simulink model "building_EXAMPLE_v1"  (R2016b)
settings: Solver=ode23tb  StartTime=-building.preruntime+8760*3600  StopTime=building.runtime+8760*3600  MaxStep=600  EnableMultiTasking=on
StartFcn:
  | tic
StopFcn:
  | toc
values from neighbouring files (symbols this model uses):
  building = create_building_automatic(building, modify, import_mode, name_XML, name_EXCEL, name_PHPP, NUMBEROFZONES)    [work_EXAMPLE_v1.m]
undefined symbols (not defined in the file or in its folder): A, B, C, cp, Dd, Dreifach, FluidMix, get_building, ID, MassFlow, p, Pressure, Qdot_C, Qdot_C_energy, Qdot_H, Qdot_H_energy, Qdot_I_electricity, Qdot_I_electricity_energy, Qdot_I_light, Qdot_I_light_energy, Qdot_I_person, Qdot_I_person_energy, Qdot_S, Qdot_S_energy, Qdot_T_ground, Qdot_T_ground_energy, Qdot_T_neighbour, Qdot_T_neighbour_energy, Qdot_T_opaque, Qdot_T_opaque_energy, Qdot_T_window, Qdot_T_window_energy, Qdot_V_infiltration, Qdot_V_infiltration_energy, Qdot_V_mech, Qdot_V_mech_energy, Qdot_V_window, Qdot_V_window_energy, rho, Tc, Temperature, Tr, Ts, Wärmeschutzglas, x_CO2, x_H2O, x_VOC
libraries: carnotUIBK x1931, carnot x83, simulink_extras x22, simulink x12
(part 10 of 35)

== system building_EXAMPLE_v1/DATALOGGER/z2 ==
  BDB : Inport
  BDB_initialize : carnotUIBK/room_node/EMPTY/BDB_initialize
  Bus Assignment : BusAssignment  AssignedSignals=Qdot_T_opaque,Qdot_T_ground,Qdot_T_neighbour,Qdot_T_window,Qdot_V_mech,Qdot_V_window,Qdot_V_infiltration,Qdot_S,Qdot_I_person,Qdot_I_light,Qdot_I_electricity,Qdot_H,Qdot_C
  Bus Selector1 : BusSelector  OutputSignals=Qdot_T_opaque,Qdot_T_ground,Qdot_T_neighbour,Qdot_T_window,Qdot_V_mech,Qdot_V_window,Qdot_V_infiltration,Qdot_S,Qdot_I_person,Qdot_I_light,Qdot_I_electricity,Qdot_H,Qdot_C
  BDB' : Outport
  wires:
  Bus Selector1/2 -> Bus Assignment/3  "<Qdot_T_ground>"
  Bus Selector1/3 -> Bus Assignment/4  "<Qdot_T_neighbour>"
  Bus Selector1/4 -> Bus Assignment/5  "<Qdot_T_window>"
  Bus Selector1/5 -> Bus Assignment/6  "<Qdot_V_mech>"
  Bus Selector1/6 -> Bus Assignment/7  "<Qdot_V_window>"
  Bus Selector1/7 -> Bus Assignment/8  "<Qdot_V_infiltration>"
  Bus Selector1/8 -> Bus Assignment/9  "<Qdot_S>"
  Bus Selector1/9 -> Bus Assignment/10  "<Qdot_I_person>"
  Bus Selector1/10 -> Bus Assignment/11  "<Qdot_I_light>"
  Bus Selector1/11 -> Bus Assignment/12  "<Qdot_I_electricity>"
  Bus Selector1/12 -> Bus Assignment/13  "<Qdot_H>"
  Bus Selector1/13 -> Bus Assignment/14  "<Qdot_C>"
  Bus Selector1/1 -> Bus Assignment/2  "<Qdot_T_opaque>"
  BDB_initialize/1 -> Bus Assignment/1
  Bus Assignment/1 -> BDB'/1
  BDB/1 -> Bus Selector1/1

== system building_EXAMPLE_v1/DATALOGGER/z3 ==
  BDB : Inport
  BDB_initialize : carnotUIBK/room_node/EMPTY/BDB_initialize
  Bus Assignment : BusAssignment  AssignedSignals=Qdot_T_opaque,Qdot_T_ground,Qdot_T_neighbour,Qdot_T_window,Qdot_V_mech,Qdot_V_window,Qdot_V_infiltration,Qdot_S,Qdot_I_person,Qdot_I_light,Qdot_I_electricity,Qdot_H,Qdot_C
  Bus Selector1 : BusSelector  OutputSignals=Qdot_T_opaque,Qdot_T_ground,Qdot_T_neighbour,Qdot_T_window,Qdot_V_mech,Qdot_V_window,Qdot_V_infiltration,Qdot_S,Qdot_I_person,Qdot_I_light,Qdot_I_electricity,Qdot_H,Qdot_C
  BDB' : Outport
  wires:
  BDB/1 -> Bus Selector1/1
  Bus Assignment/1 -> BDB'/1
  BDB_initialize/1 -> Bus Assignment/1
  Bus Selector1/1 -> Bus Assignment/2  "<Qdot_T_opaque>"
  Bus Selector1/13 -> Bus Assignment/14  "<Qdot_C>"
  Bus Selector1/12 -> Bus Assignment/13  "<Qdot_H>"
  Bus Selector1/11 -> Bus Assignment/12  "<Qdot_I_electricity>"
  Bus Selector1/10 -> Bus Assignment/11  "<Qdot_I_light>"
  Bus Selector1/9 -> Bus Assignment/10  "<Qdot_I_person>"
  Bus Selector1/8 -> Bus Assignment/9  "<Qdot_S>"
  Bus Selector1/7 -> Bus Assignment/8  "<Qdot_V_infiltration>"
  Bus Selector1/6 -> Bus Assignment/7  "<Qdot_V_window>"
  Bus Selector1/5 -> Bus Assignment/6  "<Qdot_V_mech>"
  Bus Selector1/4 -> Bus Assignment/5  "<Qdot_T_window>"
  Bus Selector1/3 -> Bus Assignment/4  "<Qdot_T_neighbour>"
  Bus Selector1/2 -> Bus Assignment/3  "<Qdot_T_ground>"

== system building_EXAMPLE_v1/DATALOGGER/z4 ==
  BDB : Inport
  BDB_initialize : carnotUIBK/room_node/EMPTY/BDB_initialize
  Bus Assignment : BusAssignment  AssignedSignals=Qdot_T_opaque,Qdot_T_ground,Qdot_T_neighbour,Qdot_T_window,Qdot_V_mech,Qdot_V_window,Qdot_V_infiltration,Qdot_S,Qdot_I_person,Qdot_I_light,Qdot_I_electricity,Qdot_H,Qdot_C
  Bus Selector1 : BusSelector  OutputSignals=Qdot_T_opaque,Qdot_T_ground,Qdot_T_neighbour,Qdot_T_window,Qdot_V_mech,Qdot_V_window,Qdot_V_infiltration,Qdot_S,Qdot_I_person,Qdot_I_light,Qdot_I_electricity,Qdot_H,Qdot_C
  BDB' : Outport
  wires:
  Bus Selector1/2 -> Bus Assignment/3  "<Qdot_T_ground>"
  Bus Selector1/3 -> Bus Assignment/4  "<Qdot_T_neighbour>"
  Bus Selector1/4 -> Bus Assignment/5  "<Qdot_T_window>"
  Bus Selector1/5 -> Bus Assignment/6  "<Qdot_V_mech>"
  Bus Selector1/6 -> Bus Assignment/7  "<Qdot_V_window>"
  Bus Selector1/7 -> Bus Assignment/8  "<Qdot_V_infiltration>"
  Bus Selector1/8 -> Bus Assignment/9  "<Qdot_S>"
  Bus Selector1/9 -> Bus Assignment/10  "<Qdot_I_person>"
  Bus Selector1/10 -> Bus Assignment/11  "<Qdot_I_light>"
  Bus Selector1/11 -> Bus Assignment/12  "<Qdot_I_electricity>"
  Bus Selector1/12 -> Bus Assignment/13  "<Qdot_H>"
  Bus Selector1/13 -> Bus Assignment/14  "<Qdot_C>"
  Bus Selector1/1 -> Bus Assignment/2  "<Qdot_T_opaque>"
  BDB_initialize/1 -> Bus Assignment/1
  Bus Assignment/1 -> BDB'/1
  BDB/1 -> Bus Selector1/1

== system building_EXAMPLE_v1/DATALOGGER/z5 ==
  BDB : Inport
  BDB_initialize : carnotUIBK/room_node/EMPTY/BDB_initialize
  Bus Assignment : BusAssignment  AssignedSignals=Qdot_T_opaque,Qdot_T_ground,Qdot_T_neighbour,Qdot_T_window,Qdot_V_mech,Qdot_V_window,Qdot_V_infiltration,Qdot_S,Qdot_I_person,Qdot_I_light,Qdot_I_electricity,Qdot_H,Qdot_C
  Bus Selector1 : BusSelector  OutputSignals=Qdot_T_opaque,Qdot_T_ground,Qdot_T_neighbour,Qdot_T_window,Qdot_V_mech,Qdot_V_window,Qdot_V_infiltration,Qdot_S,Qdot_I_person,Qdot_I_light,Qdot_I_electricity,Qdot_H,Qdot_C
  BDB' : Outport
  wires:
  BDB/1 -> Bus Selector1/1
  Bus Assignment/1 -> BDB'/1
  BDB_initialize/1 -> Bus Assignment/1
  Bus Selector1/1 -> Bus Assignment/2  "<Qdot_T_opaque>"
  Bus Selector1/13 -> Bus Assignment/14  "<Qdot_C>"
  Bus Selector1/12 -> Bus Assignment/13  "<Qdot_H>"
  Bus Selector1/11 -> Bus Assignment/12  "<Qdot_I_electricity>"
  Bus Selector1/10 -> Bus Assignment/11  "<Qdot_I_light>"
  Bus Selector1/9 -> Bus Assignment/10  "<Qdot_I_person>"
  Bus Selector1/8 -> Bus Assignment/9  "<Qdot_S>"
  Bus Selector1/7 -> Bus Assignment/8  "<Qdot_V_infiltration>"
  Bus Selector1/6 -> Bus Assignment/7  "<Qdot_V_window>"
  Bus Selector1/5 -> Bus Assignment/6  "<Qdot_V_mech>"
  Bus Selector1/4 -> Bus Assignment/5  "<Qdot_T_window>"
  Bus Selector1/3 -> Bus Assignment/4  "<Qdot_T_neighbour>"
  Bus Selector1/2 -> Bus Assignment/3  "<Qdot_T_ground>"

== system building_EXAMPLE_v1/DATALOGGER/z6 ==
  BDB : Inport
  BDB_initialize : carnotUIBK/room_node/EMPTY/BDB_initialize
  Bus Assignment : BusAssignment  AssignedSignals=Qdot_T_opaque,Qdot_T_ground,Qdot_T_neighbour,Qdot_T_window,Qdot_V_mech,Qdot_V_window,Qdot_V_infiltration,Qdot_S,Qdot_I_person,Qdot_I_light,Qdot_I_electricity,Qdot_H,Qdot_C
  Bus Selector1 : BusSelector  OutputSignals=Qdot_T_opaque,Qdot_T_ground,Qdot_T_neighbour,Qdot_T_window,Qdot_V_mech,Qdot_V_window,Qdot_V_infiltration,Qdot_S,Qdot_I_person,Qdot_I_light,Qdot_I_electricity,Qdot_H,Qdot_C
  BDB' : Outport
  wires:
  Bus Selector1/2 -> Bus Assignment/3  "<Qdot_T_ground>"
  Bus Selector1/3 -> Bus Assignment/4  "<Qdot_T_neighbour>"
  Bus Selector1/4 -> Bus Assignment/5  "<Qdot_T_window>"
  Bus Selector1/5 -> Bus Assignment/6  "<Qdot_V_mech>"
  Bus Selector1/6 -> Bus Assignment/7  "<Qdot_V_window>"
  Bus Selector1/7 -> Bus Assignment/8  "<Qdot_V_infiltration>"
  Bus Selector1/8 -> Bus Assignment/9  "<Qdot_S>"
  Bus Selector1/9 -> Bus Assignment/10  "<Qdot_I_person>"
  Bus Selector1/10 -> Bus Assignment/11  "<Qdot_I_light>"
  Bus Selector1/11 -> Bus Assignment/12  "<Qdot_I_electricity>"
  Bus Selector1/12 -> Bus Assignment/13  "<Qdot_H>"
  Bus Selector1/13 -> Bus Assignment/14  "<Qdot_C>"
  Bus Selector1/1 -> Bus Assignment/2  "<Qdot_T_opaque>"
  BDB_initialize/1 -> Bus Assignment/1
  Bus Assignment/1 -> BDB'/1
  BDB/1 -> Bus Selector1/1

== system building_EXAMPLE_v1/DATALOGGER/z7 ==
  BDB : Inport
  BDB_initialize : carnotUIBK/room_node/EMPTY/BDB_initialize
  Bus Assignment : BusAssignment  AssignedSignals=Qdot_T_opaque,Qdot_T_ground,Qdot_T_neighbour,Qdot_T_window,Qdot_V_mech,Qdot_V_window,Qdot_V_infiltration,Qdot_S,Qdot_I_person,Qdot_I_light,Qdot_I_electricity,Qdot_H,Qdot_C
  Bus Selector1 : BusSelector  OutputSignals=Qdot_T_opaque,Qdot_T_ground,Qdot_T_neighbour,Qdot_T_window,Qdot_V_mech,Qdot_V_window,Qdot_V_infiltration,Qdot_S,Qdot_I_person,Qdot_I_light,Qdot_I_electricity,Qdot_H,Qdot_C
  BDB' : Outport
  wires:
  BDB/1 -> Bus Selector1/1
  Bus Assignment/1 -> BDB'/1
  BDB_initialize/1 -> Bus Assignment/1
  Bus Selector1/1 -> Bus Assignment/2  "<Qdot_T_opaque>"
  Bus Selector1/13 -> Bus Assignment/14  "<Qdot_C>"
  Bus Selector1/12 -> Bus Assignment/13  "<Qdot_H>"
  Bus Selector1/11 -> Bus Assignment/12  "<Qdot_I_electricity>"
  Bus Selector1/10 -> Bus Assignment/11  "<Qdot_I_light>"
  Bus Selector1/9 -> Bus Assignment/10  "<Qdot_I_person>"
  Bus Selector1/8 -> Bus Assignment/9  "<Qdot_S>"
  Bus Selector1/7 -> Bus Assignment/8  "<Qdot_V_infiltration>"
  Bus Selector1/6 -> Bus Assignment/7  "<Qdot_V_window>"
  Bus Selector1/5 -> Bus Assignment/6  "<Qdot_V_mech>"
  Bus Selector1/4 -> Bus Assignment/5  "<Qdot_T_window>"
  Bus Selector1/3 -> Bus Assignment/4  "<Qdot_T_neighbour>"
  Bus Selector1/2 -> Bus Assignment/3  "<Qdot_T_ground>"

== system building_EXAMPLE_v1/DATALOGGER/z8 ==
  BDB : Inport
  BDB_initialize : carnotUIBK/room_node/EMPTY/BDB_initialize
  Bus Assignment : BusAssignment  AssignedSignals=Qdot_T_opaque,Qdot_T_ground,Qdot_T_neighbour,Qdot_T_window,Qdot_V_mech,Qdot_V_window,Qdot_V_infiltration,Qdot_S,Qdot_I_person,Qdot_I_light,Qdot_I_electricity,Qdot_H,Qdot_C
  Bus Selector1 : BusSelector  OutputSignals=Qdot_T_opaque,Qdot_T_ground,Qdot_T_neighbour,Qdot_T_window,Qdot_V_mech,Qdot_V_window,Qdot_V_infiltration,Qdot_S,Qdot_I_person,Qdot_I_light,Qdot_I_electricity,Qdot_H,Qdot_C
  BDB' : Outport
  wires:
  Bus Selector1/2 -> Bus Assignment/3  "<Qdot_T_ground>"
  Bus Selector1/3 -> Bus Assignment/4  "<Qdot_T_neighbour>"
  Bus Selector1/4 -> Bus Assignment/5  "<Qdot_T_window>"
  Bus Selector1/5 -> Bus Assignment/6  "<Qdot_V_mech>"
  Bus Selector1/6 -> Bus Assignment/7  "<Qdot_V_window>"
  Bus Selector1/7 -> Bus Assignment/8  "<Qdot_V_infiltration>"
  Bus Selector1/8 -> Bus Assignment/9  "<Qdot_S>"
  Bus Selector1/9 -> Bus Assignment/10  "<Qdot_I_person>"
  Bus Selector1/10 -> Bus Assignment/11  "<Qdot_I_light>"
  Bus Selector1/11 -> Bus Assignment/12  "<Qdot_I_electricity>"
  Bus Selector1/12 -> Bus Assignment/13  "<Qdot_H>"
  Bus Selector1/13 -> Bus Assignment/14  "<Qdot_C>"
  Bus Selector1/1 -> Bus Assignment/2  "<Qdot_T_opaque>"
  BDB_initialize/1 -> Bus Assignment/1
  Bus Assignment/1 -> BDB'/1
  BDB/1 -> Bus Selector1/1

== system building_EXAMPLE_v1/DATALOGGER/z9 ==
  BDB : Inport
  BDB_initialize : carnotUIBK/room_node/EMPTY/BDB_initialize
  Bus Assignment : BusAssignment  AssignedSignals=Qdot_T_opaque,Qdot_T_ground,Qdot_T_neighbour,Qdot_T_window,Qdot_V_mech,Qdot_V_window,Qdot_V_infiltration,Qdot_S,Qdot_I_person,Qdot_I_light,Qdot_I_electricity,Qdot_H,Qdot_C
  Bus Selector1 : BusSelector  OutputSignals=Qdot_T_opaque,Qdot_T_ground,Qdot_T_neighbour,Qdot_T_window,Qdot_V_mech,Qdot_V_window,Qdot_V_infiltration,Qdot_S,Qdot_I_person,Qdot_I_light,Qdot_I_electricity,Qdot_H,Qdot_C
  BDB' : Outport
  wires:
  BDB/1 -> Bus Selector1/1
  Bus Assignment/1 -> BDB'/1
  BDB_initialize/1 -> Bus Assignment/1
  Bus Selector1/1 -> Bus Assignment/2  "<Qdot_T_opaque>"
  Bus Selector1/13 -> Bus Assignment/14  "<Qdot_C>"
  Bus Selector1/12 -> Bus Assignment/13  "<Qdot_H>"
  Bus Selector1/11 -> Bus Assignment/12  "<Qdot_I_electricity>"
  Bus Selector1/10 -> Bus Assignment/11  "<Qdot_I_light>"
  Bus Selector1/9 -> Bus Assignment/10  "<Qdot_I_person>"
  Bus Selector1/8 -> Bus Assignment/9  "<Qdot_S>"
  Bus Selector1/7 -> Bus Assignment/8  "<Qdot_V_infiltration>"
  Bus Selector1/6 -> Bus Assignment/7  "<Qdot_V_window>"
  Bus Selector1/5 -> Bus Assignment/6  "<Qdot_V_mech>"
  Bus Selector1/4 -> Bus Assignment/5  "<Qdot_T_window>"
  Bus Selector1/3 -> Bus Assignment/4  "<Qdot_T_neighbour>"
  Bus Selector1/2 -> Bus Assignment/3  "<Qdot_T_ground>"

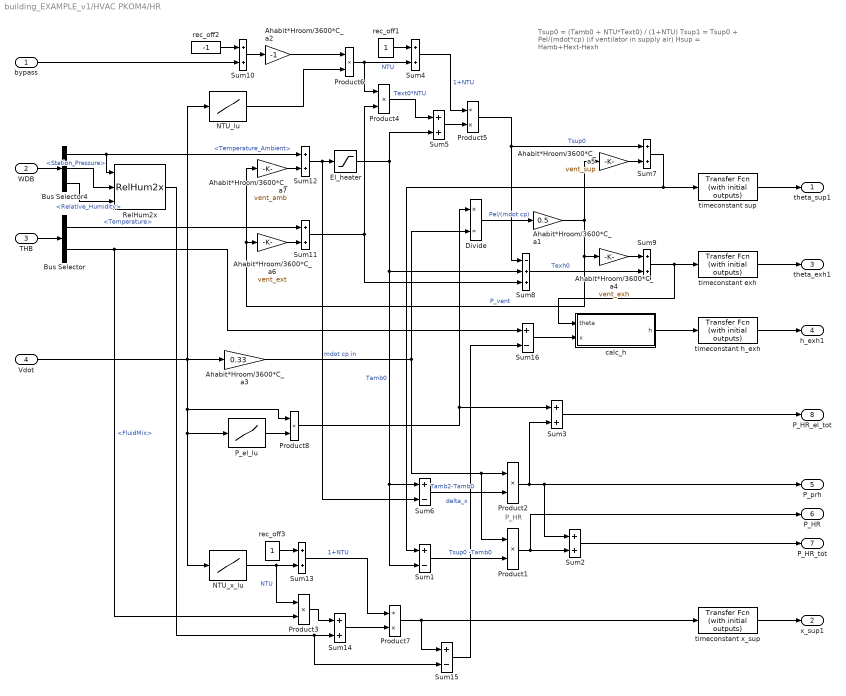
== system building_EXAMPLE_v1/HVAC PKOM4/HR ==
  note: P_HR
  note: Tsup0 = (Tamb0 + NTU*Text0) / (1+NTU)
      | Tsup1 = Tsup0 + Pel/(mdot*cp)  (if ventilator in supply air)
      | Hsup = Hamb+Hext-Hexh
  bypass : Inport
  WDB : Inport  Port=2
  THB : Inport  Port=3
  Vdot : Inport  Port=4
  Ahabit*Hroom/3600*C_a1 : Gain  Gain=0.5  SaturateOnIntegerOverflow=on  OutDataTypeStr=Inherit: Same as input  ParamDataTypeStr=Inherit: Same as input
  Ahabit*Hroom/3600*C_a2 : Gain  Gain=-1  SaturateOnIntegerOverflow=on  OutDataTypeStr=Inherit: Same as input  ParamDataTypeStr=Inherit: Same as input
  Ahabit*Hroom/3600*C_a3 : Gain  Gain=0.33  SaturateOnIntegerOverflow=on  OutDataTypeStr=Inherit: Same as input  ParamDataTypeStr=Inherit: Same as input
  Ahabit*Hroom/3600*C_a4 : Gain  Gain=vent_exh  SaturateOnIntegerOverflow=on  OutDataTypeStr=Inherit: Same as input  ParamDataTypeStr=Inherit: Same as input
  Ahabit*Hroom/3600*C_a5 : Gain  Gain=vent_sup  SaturateOnIntegerOverflow=on  OutDataTypeStr=Inherit: Same as input  ParamDataTypeStr=Inherit: Same as input
  Ahabit*Hroom/3600*C_a6 : Gain  Gain=vent_ext  SaturateOnIntegerOverflow=on  OutDataTypeStr=Inherit: Same as input  ParamDataTypeStr=Inherit: Same as input
  Ahabit*Hroom/3600*C_a7 : Gain  Gain=vent_amb  SaturateOnIntegerOverflow=on  OutDataTypeStr=Inherit: Same as input  ParamDataTypeStr=Inherit: Same as input
  Bus Selector : BusSelector  OutputSignals=Temperature,FluidMix
  Bus Selector4 : BusSelector  OutputSignals=Temperature_Ambient,Station_Pressure,Relative_Humidity
  Divide : Product  Inputs=*/
  El_heater : Saturate  UpperLimit=inf  LowerLimit=low_lim
  NTU_lu : Lookup_n-D  NumberOfTableDimensions=1  BreakpointsForDimension1=Vdot  Table=NTU  InternalRulePriority=Speed  RndMeth=Simplest  InputSameDT=on
  NTU_x_lu : Lookup_n-D  NumberOfTableDimensions=1  BreakpointsForDimension1=Vdot  Table=NTU_x  InternalRulePriority=Speed  RndMeth=Simplest  InputSameDT=on
  P_el_lu : Lookup_n-D  NumberOfTableDimensions=1  BreakpointsForDimension1=Vdot  Table=p_el  InternalRulePriority=Speed  RndMeth=Simplest  InputSameDT=on
  Product{1..4,6,8} (6 alike) : Product  SaturateOnIntegerOverflow=on  InputSameDT=on  OutDataTypeStr=Inherit: Same as first input
  Product5 : Product  Inputs=/*  SaturateOnIntegerOverflow=on  InputSameDT=on  OutDataTypeStr=Inherit: Same as first input
  Product7 : Product  Inputs=/*  SaturateOnIntegerOverflow=on  InputSameDT=on  OutDataTypeStr=Inherit: Same as first input
  RelHum2x : carnot/Basic/Material_Properties/RelHum2x
  Sum{1,6,15..16} (4 alike) : Sum  Inputs=+-  SaturateOnIntegerOverflow=on  InputSameDT=on  OutDataTypeStr=Inherit: Same as first input
  Sum{4..5,7,9..14} (9 alike) : Sum  Inputs=2  SaturateOnIntegerOverflow=on  InputSameDT=on  OutDataTypeStr=Inherit: Same as first input
  Sum2 : Sum  SaturateOnIntegerOverflow=on  InputSameDT=on  OutDataTypeStr=Inherit: Same as first input
  Sum3 : Sum  SaturateOnIntegerOverflow=on  InputSameDT=on  OutDataTypeStr=Inherit: Same as first input
  Sum8 : Sum  Inputs=-++  SaturateOnIntegerOverflow=on  InputSameDT=on  OutDataTypeStr=Inherit: Same as first input
  calc_h : Subsystem
  rec_off1 : Constant
  rec_off2 : Constant  Value=-1
  rec_off3 : Constant
  timeconstant exh : simulink_extras/Additional Linear/Transfer Fcn (with initial outputs)  N=[1]  D=[120 1]  Y0=0  U0=0
  timeconstant h_exh : simulink_extras/Additional Linear/Transfer Fcn (with initial outputs)  N=[1]  D=[120 1]  Y0=0  U0=0
  timeconstant sup : simulink_extras/Additional Linear/Transfer Fcn (with initial outputs)  N=[1]  D=[120 1]  Y0=20  U0=0
  timeconstant x_sup : simulink_extras/Additional Linear/Transfer Fcn (with initial outputs)  N=[1]  D=[120 1]  Y0=0  U0=0
  theta_sup1 : Outport
  x_sup1 : Outport  Port=2
  theta_exh1 : Outport  Port=3
  h_exh1 : Outport  Port=4
  P_prh : Outport  Port=5
  P_HR : Outport  Port=6
  P_HR_tot : Outport  Port=7
  P_HR_el_tot : Outport  Port=8
  wires:
  P_el_lu/1 -> Product8/2
  timeconstant x_sup/1 -> x_sup1/1
  timeconstant h_exh/1 -> h_exh1/1
  timeconstant exh/1 -> theta_exh1/1
  timeconstant sup/1 -> theta_sup1/1
  Sum16/1 -> calc_h/2(x)
  Sum15/1 -> Sum16/2  "delta_x"
  Product7/1 -> Sum15/1, timeconstant x_sup/1
  Sum14/1 -> Product7/2
  Product3/1 -> Sum14/1
  NTU_x_lu/1 -> Sum13/2, Product3/1  "NTU"
  Sum13/1 -> Product7/1  "1+NTU"
  rec_off3/1 -> Sum13/1
  Bus Selector4/3 -> RelHum2x/3  "<Relative_Humidity>"
  Bus Selector4/2 -> RelHum2x/2  "<Station_Pressure>"
  RelHum2x/1 -> Sum14/2, Sum15/2
  Sum6/1 -> Product2/2  "Tamb2-Tamb0"
  Sum9/1 -> calc_h/1(theta), timeconstant exh/1
  Sum11/1 -> Sum8/3, Product4/2
  Vdot/1 -> Ahabit*Hroom/3600*C_a3/1, NTU_lu/1, NTU_x_lu/1, P_el_lu/1, Product8/1
  Sum7/1 -> timeconstant sup/1, Sum1/1
  El_heater/1 -> Sum5/2, Sum6/1, Sum1/2, Sum8/2  "Tamb0"
  Product2/1 -> P_prh/1, Sum2/1, Sum3/2
  Sum1/1 -> Product1/2  "Tsup0 -Tamb0"
  Product1/1 -> Sum2/2, P_HR/1
  Sum2/1 -> P_HR_tot/1
  Sum3/1 -> P_HR_el_tot/1
  Product6/1 -> Product4/1, Sum4/2  "NTU"
  NTU_lu/1 -> Product6/2
  Sum4/1 -> Product5/1  "1+NTU"
  Product4/1 -> Sum5/1  "Text0*NTU"
  rec_off1/1 -> Sum4/1
  Sum5/1 -> Product5/2
  Product5/1 -> Sum7/1, Sum8/1  "Tsup0"
  Divide/1 -> Ahabit*Hroom/3600*C_a1/1  "Pel/(mdot cp)"
  Product8/1 -> Sum3/1, Divide/1
  Ahabit*Hroom/3600*C_a1/1 -> Ahabit*Hroom/3600*C_a5/1, Ahabit*Hroom/3600*C_a7/1, Ahabit*Hroom/3600*C_a6/1, Ahabit*Hroom/3600*C_a4/1  "P_vent"
  Sum8/1 -> Sum9/2  "Texh0"
  Ahabit*Hroom/3600*C_a3/1 -> Divide/2, Product2/1, Product1/1  "mdot cp in"
  Ahabit*Hroom/3600*C_a2/1 -> Product6/1
  rec_off2/1 -> Sum10/1
  bypass/1 -> Sum10/2
  Sum10/1 -> Ahabit*Hroom/3600*C_a2/1
  WDB/1 -> Bus Selector4/1
  Sum12/1 -> El_heater/1, Sum6/2
  THB/1 -> Bus Selector/1
  Ahabit*Hroom/3600*C_a4/1 -> Sum9/1
  Ahabit*Hroom/3600*C_a5/1 -> Sum7/2
  calc_h/1(h) -> timeconstant h_exh/1
  Bus Selector/2 -> Product3/2, Sum16/1  "<FluidMix>"
  Ahabit*Hroom/3600*C_a6/1 -> Sum11/2
  Bus Selector/1 -> Sum11/1  "<Temperature>"
  Ahabit*Hroom/3600*C_a7/1 -> Sum12/2
  Bus Selector4/1 -> Sum12/1, RelHum2x/1  "<Temperature_Ambient>"

== system building_EXAMPLE_v1/HVAC PKOM4/HR unit ==
  note: P_HR
  note: Tsup0 = (Tamb0 + NTU*Text0) / (1+NTU)
      | Tsup1 = Tsup0 + Pel/(mdot*cp)  (if ventilator in supply air)
      | Hsup = Hamb+Hext-Hexh
  bypass : Inport
  WDB : Inport  Port=2
  THB : Inport  Port=3
  Vdot : Inport  Port=4
  Ahabit*Hroom/3600*C_a1 : Gain  Gain=0.5  SaturateOnIntegerOverflow=on  OutDataTypeStr=Inherit: Same as input  ParamDataTypeStr=Inherit: Same as input
  Ahabit*Hroom/3600*C_a2 : Gain  Gain=-1  SaturateOnIntegerOverflow=on  OutDataTypeStr=Inherit: Same as input  ParamDataTypeStr=Inherit: Same as input
  Ahabit*Hroom/3600*C_a3 : Gain  Gain=cp_a * rho_a / 3600  SaturateOnIntegerOverflow=on  OutDataTypeStr=Inherit: Same as input  ParamDataTypeStr=Inherit: Same as input
  Ahabit*Hroom/3600*C_a4 : Gain  Gain=vent_exh  SaturateOnIntegerOverflow=on  OutDataTypeStr=Inherit: Same as input  ParamDataTypeStr=Inherit: Same as input
  Ahabit*Hroom/3600*C_a5 : Gain  Gain=vent_sup  SaturateOnIntegerOverflow=on  OutDataTypeStr=Inherit: Same as input  ParamDataTypeStr=Inherit: Same as input
  Ahabit*Hroom/3600*C_a6 : Gain  Gain=vent_ext  SaturateOnIntegerOverflow=on  OutDataTypeStr=Inherit: Same as input  ParamDataTypeStr=Inherit: Same as input
  Ahabit*Hroom/3600*C_a7 : Gain  Gain=vent_amb  SaturateOnIntegerOverflow=on  OutDataTypeStr=Inherit: Same as input  ParamDataTypeStr=Inherit: Same as input
  Bus Selector : BusSelector  OutputSignals=Temperature,FluidMix
  Bus Selector4 : BusSelector  OutputSignals=Temperature_Ambient,Station_Pressure,Relative_Humidity
  Divide : Product  Inputs=*/
  El_heater : Saturate  UpperLimit=inf  LowerLimit=low_lim
  NTU : Constant  Value=NTU
  Product{1..2,4,6} (4 alike) : Product  SaturateOnIntegerOverflow=on  InputSameDT=on  OutDataTypeStr=Inherit: Same as first input
  Product5 : Product  Inputs=/*  SaturateOnIntegerOverflow=on  InputSameDT=on  OutDataTypeStr=Inherit: Same as first input
  RelHum2x : carnot/Basic/Material_Properties/RelHum2x
  Sum1 : Sum  Inputs=+-  SaturateOnIntegerOverflow=on  InputSameDT=on  OutDataTypeStr=Inherit: Same as first input
  Sum{4..5,7,9..12} (7 alike) : Sum  Inputs=2  SaturateOnIntegerOverflow=on  InputSameDT=on  OutDataTypeStr=Inherit: Same as first input
  Sum2 : Sum  SaturateOnIntegerOverflow=on  InputSameDT=on  OutDataTypeStr=Inherit: Same as first input
  Sum3 : Sum  SaturateOnIntegerOverflow=on  InputSameDT=on  OutDataTypeStr=Inherit: Same as first input
  Sum6 : Sum  Inputs=+-  SaturateOnIntegerOverflow=on  InputSameDT=on  OutDataTypeStr=Inherit: Same as first input
  Sum8 : Sum  Inputs=-++  SaturateOnIntegerOverflow=on  InputSameDT=on  OutDataTypeStr=Inherit: Same as first input
  calc_h : Subsystem
  rec_off1 : Constant
  rec_off2 : Constant  Value=-1
  rec_off4 : Constant  Value=P_elec
  theta_sup1 : Outport
  x_sup1 : Outport  Port=2
  theta_exh1 : Outport  Port=3
  h_exh1 : Outport  Port=4
  P_prh : Outport  Port=5
  P_HR : Outport  Port=6
  P_HR_tot : Outport  Port=7
  P_HR_el_tot : Outport  Port=8
  wires:
  Sum6/1 -> Product2/2  "Tamb2-Tamb0"
  Sum9/1 -> calc_h/1(theta), theta_exh1/1
  Sum11/1 -> Sum8/3, Product4/2
  Vdot/1 -> Ahabit*Hroom/3600*C_a3/1
  Sum7/1 -> theta_sup1/1, Sum1/1
  El_heater/1 -> Sum6/1, Sum1/2, Sum8/2, Sum5/2  "Tamb0"
  Product2/1 -> P_prh/1, Sum2/1, Sum3/2
  Sum1/1 -> Product1/2  "Tsup0 -Tamb0"
  Product1/1 -> Sum2/2, P_HR/1
  Sum2/1 -> P_HR_tot/1
  Sum3/1 -> P_HR_el_tot/1
  Product6/1 -> Product4/1, Sum4/2  "NTU"
  NTU/1 -> Product6/2
  Sum4/1 -> Product5/1  "1+NTU"
  Product4/1 -> Sum5/1  "Text0*NTU"
  rec_off1/1 -> Sum4/1
  Sum5/1 -> Product5/2
  Product5/1 -> Sum7/1, Sum8/1  "Tsup0"
  Divide/1 -> Ahabit*Hroom/3600*C_a1/1  "Pel/(mdot cp)"
  rec_off4/1 -> Sum3/1, Divide/1
  Ahabit*Hroom/3600*C_a1/1 -> Ahabit*Hroom/3600*C_a5/1, Ahabit*Hroom/3600*C_a7/1, Ahabit*Hroom/3600*C_a6/1, Ahabit*Hroom/3600*C_a4/1  "P_vent"
  Sum8/1 -> Sum9/2  "Texh0"
  Ahabit*Hroom/3600*C_a3/1 -> Divide/2, Product2/1, Product1/1  "mdot cp in"
  Ahabit*Hroom/3600*C_a2/1 -> Product6/1
  rec_off2/1 -> Sum10/1
  bypass/1 -> Sum10/2
  Sum10/1 -> Ahabit*Hroom/3600*C_a2/1
  WDB/1 -> Bus Selector4/1
  Sum12/1 -> El_heater/1, Sum6/2
  THB/1 -> Bus Selector/1
  Ahabit*Hroom/3600*C_a4/1 -> Sum9/1
  Ahabit*Hroom/3600*C_a5/1 -> Sum7/2
  calc_h/1(h) -> h_exh1/1
  Bus Selector/2 -> calc_h/2(x)  "<FluidMix>"
  Ahabit*Hroom/3600*C_a6/1 -> Sum11/2
  Bus Selector/1 -> Sum11/1  "<Temperature>"
  Ahabit*Hroom/3600*C_a7/1 -> Sum12/2
  Bus Selector4/1 -> Sum12/1, RelHum2x/1  "<Temperature_Ambient>"
  Bus Selector4/2 -> RelHum2x/2  "<Station_Pressure>"
  Bus Selector4/3 -> RelHum2x/3  "<Relative_Humidity>"
  RelHum2x/1 -> x_sup1/1

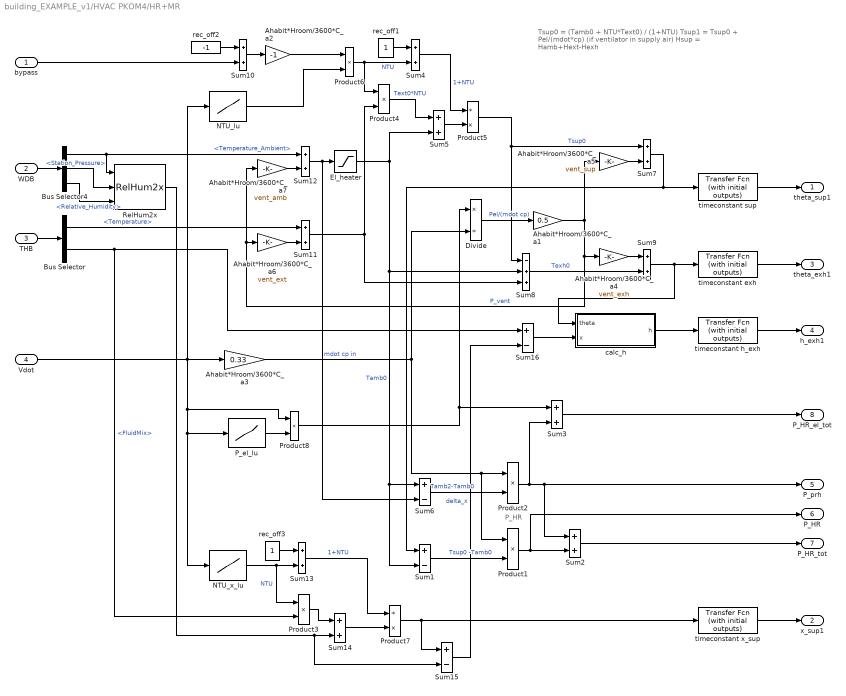
== system building_EXAMPLE_v1/HVAC PKOM4/HR+MR ==
  note: Tsup0 = (Tamb0 + NTU*Text0) / (1+NTU)
      | Tsup1 = Tsup0 + Pel/(mdot*cp)  (if ventilator in supply air)
      | Hsup = Hamb+Hext-Hexh
  note: P_HR
  bypass : Inport
  WDB : Inport  Port=2
  THB : Inport  Port=3
  Vdot : Inport  Port=4
  Ahabit*Hroom/3600*C_a1 : Gain  Gain=0.5  SaturateOnIntegerOverflow=on  OutDataTypeStr=Inherit: Same as input  ParamDataTypeStr=Inherit: Same as input
  Ahabit*Hroom/3600*C_a2 : Gain  Gain=-1  SaturateOnIntegerOverflow=on  OutDataTypeStr=Inherit: Same as input  ParamDataTypeStr=Inherit: Same as input
  Ahabit*Hroom/3600*C_a3 : Gain  Gain=0.33  SaturateOnIntegerOverflow=on  OutDataTypeStr=Inherit: Same as input  ParamDataTypeStr=Inherit: Same as input
  Ahabit*Hroom/3600*C_a4 : Gain  Gain=vent_exh  SaturateOnIntegerOverflow=on  OutDataTypeStr=Inherit: Same as input  ParamDataTypeStr=Inherit: Same as input
  Ahabit*Hroom/3600*C_a5 : Gain  Gain=vent_sup  SaturateOnIntegerOverflow=on  OutDataTypeStr=Inherit: Same as input  ParamDataTypeStr=Inherit: Same as input
  Ahabit*Hroom/3600*C_a6 : Gain  Gain=vent_ext  SaturateOnIntegerOverflow=on  OutDataTypeStr=Inherit: Same as input  ParamDataTypeStr=Inherit: Same as input
  Ahabit*Hroom/3600*C_a7 : Gain  Gain=vent_amb  SaturateOnIntegerOverflow=on  OutDataTypeStr=Inherit: Same as input  ParamDataTypeStr=Inherit: Same as input
  Bus Selector : BusSelector  OutputSignals=Temperature,FluidMix
  Bus Selector4 : BusSelector  OutputSignals=Temperature_Ambient,Station_Pressure,Relative_Humidity
  Divide : Product  Inputs=*/
  El_heater : Saturate  UpperLimit=inf  LowerLimit=low_lim
  NTU_lu : Lookup_n-D  NumberOfTableDimensions=1  BreakpointsForDimension1=Vdot  Table=NTU  InternalRulePriority=Speed  RndMeth=Simplest  InputSameDT=on
  NTU_x_lu : Lookup_n-D  NumberOfTableDimensions=1  BreakpointsForDimension1=Vdot  Table=NTU_x  InternalRulePriority=Speed  RndMeth=Simplest  InputSameDT=on
  P_el_lu : Lookup_n-D  NumberOfTableDimensions=1  BreakpointsForDimension1=Vdot  Table=p_el  InternalRulePriority=Speed  RndMeth=Simplest  InputSameDT=on
  Product{1..4,6,8} (6 alike) : Product  SaturateOnIntegerOverflow=on  InputSameDT=on  OutDataTypeStr=Inherit: Same as first input
  Product5 : Product  Inputs=/*  SaturateOnIntegerOverflow=on  InputSameDT=on  OutDataTypeStr=Inherit: Same as first input
  Product7 : Product  Inputs=/*  SaturateOnIntegerOverflow=on  InputSameDT=on  OutDataTypeStr=Inherit: Same as first input
  RelHum2x : carnot/Basic/Material_Properties/RelHum2x
  Sum{1,6,15..16} (4 alike) : Sum  Inputs=+-  SaturateOnIntegerOverflow=on  InputSameDT=on  OutDataTypeStr=Inherit: Same as first input
  Sum{4..5,7,9..14} (9 alike) : Sum  Inputs=2  SaturateOnIntegerOverflow=on  InputSameDT=on  OutDataTypeStr=Inherit: Same as first input
  Sum2 : Sum  SaturateOnIntegerOverflow=on  InputSameDT=on  OutDataTypeStr=Inherit: Same as first input
  Sum3 : Sum  SaturateOnIntegerOverflow=on  InputSameDT=on  OutDataTypeStr=Inherit: Same as first input
  Sum8 : Sum  Inputs=-++  SaturateOnIntegerOverflow=on  InputSameDT=on  OutDataTypeStr=Inherit: Same as first input
  calc_h : Subsystem
  rec_off1 : Constant
  rec_off2 : Constant  Value=-1
  rec_off3 : Constant
  timeconstant exh : simulink_extras/Additional Linear/Transfer Fcn (with initial outputs)  N=[1]  D=[120 1]  Y0=0  U0=0
  timeconstant h_exh : simulink_extras/Additional Linear/Transfer Fcn (with initial outputs)  N=[1]  D=[120 1]  Y0=0  U0=0
  timeconstant sup : simulink_extras/Additional Linear/Transfer Fcn (with initial outputs)  N=[1]  D=[120 1]  Y0=20  U0=0
  timeconstant x_sup : simulink_extras/Additional Linear/Transfer Fcn (with initial outputs)  N=[1]  D=[120 1]  Y0=0  U0=0
  theta_sup1 : Outport
  x_sup1 : Outport  Port=2
  theta_exh1 : Outport  Port=3
  h_exh1 : Outport  Port=4
  P_prh : Outport  Port=5
  P_HR : Outport  Port=6
  P_HR_tot : Outport  Port=7
  P_HR_el_tot : Outport  Port=8
  wires:
  Bus Selector4/1 -> RelHum2x/1, Sum12/1  "<Temperature_Ambient>"
  Ahabit*Hroom/3600*C_a7/1 -> Sum12/2
  Bus Selector/1 -> Sum11/1  "<Temperature>"
  Ahabit*Hroom/3600*C_a6/1 -> Sum11/2
  Bus Selector/2 -> Sum16/1, Product3/2  "<FluidMix>"
  calc_h/1(h) -> timeconstant h_exh/1
  Ahabit*Hroom/3600*C_a5/1 -> Sum7/2
  Ahabit*Hroom/3600*C_a4/1 -> Sum9/1
  THB/1 -> Bus Selector/1
  Sum12/1 -> Sum6/2, El_heater/1
  WDB/1 -> Bus Selector4/1
  Sum10/1 -> Ahabit*Hroom/3600*C_a2/1
  bypass/1 -> Sum10/2
  rec_off2/1 -> Sum10/1
  Ahabit*Hroom/3600*C_a2/1 -> Product6/1
  Ahabit*Hroom/3600*C_a3/1 -> Product1/1, Product2/1, Divide/2  "mdot cp in"
  Sum8/1 -> Sum9/2  "Texh0"
  Ahabit*Hroom/3600*C_a1/1 -> Ahabit*Hroom/3600*C_a4/1, Ahabit*Hroom/3600*C_a6/1, Ahabit*Hroom/3600*C_a7/1, Ahabit*Hroom/3600*C_a5/1  "P_vent"
  Product8/1 -> Divide/1, Sum3/1
  Divide/1 -> Ahabit*Hroom/3600*C_a1/1  "Pel/(mdot cp)"
  Product5/1 -> Sum8/1, Sum7/1  "Tsup0"
  Sum5/1 -> Product5/2
  rec_off1/1 -> Sum4/1
  Product4/1 -> Sum5/1  "Text0*NTU"
  Sum4/1 -> Product5/1  "1+NTU"
  NTU_lu/1 -> Product6/2
  Product6/1 -> Sum4/2, Product4/1  "NTU"
  Sum3/1 -> P_HR_el_tot/1
  Sum2/1 -> P_HR_tot/1
  Product1/1 -> P_HR/1, Sum2/2
  Sum1/1 -> Product1/2  "Tsup0 -Tamb0"
  Product2/1 -> Sum3/2, Sum2/1, P_prh/1
  El_heater/1 -> Sum8/2, Sum1/2, Sum6/1, Sum5/2  "Tamb0"
  Sum7/1 -> Sum1/1, timeconstant sup/1
  Vdot/1 -> Product8/1, P_el_lu/1, NTU_x_lu/1, NTU_lu/1, Ahabit*Hroom/3600*C_a3/1
  Sum11/1 -> Product4/2, Sum8/3
  Sum9/1 -> timeconstant exh/1, calc_h/1(theta)
  Sum6/1 -> Product2/2  "Tamb2-Tamb0"
  RelHum2x/1 -> Sum15/2, Sum14/2
  Bus Selector4/2 -> RelHum2x/2  "<Station_Pressure>"
  Bus Selector4/3 -> RelHum2x/3  "<Relative_Humidity>"
  rec_off3/1 -> Sum13/1
  Sum13/1 -> Product7/1  "1+NTU"
  NTU_x_lu/1 -> Product3/1, Sum13/2  "NTU"
  Product3/1 -> Sum14/1
  Sum14/1 -> Product7/2
  Product7/1 -> timeconstant x_sup/1, Sum15/1
  Sum15/1 -> Sum16/2  "delta_x"
  Sum16/1 -> calc_h/2(x)
  timeconstant sup/1 -> theta_sup1/1
  timeconstant exh/1 -> theta_exh1/1
  timeconstant h_exh/1 -> h_exh1/1
  timeconstant x_sup/1 -> x_sup1/1
  P_el_lu/1 -> Product8/2

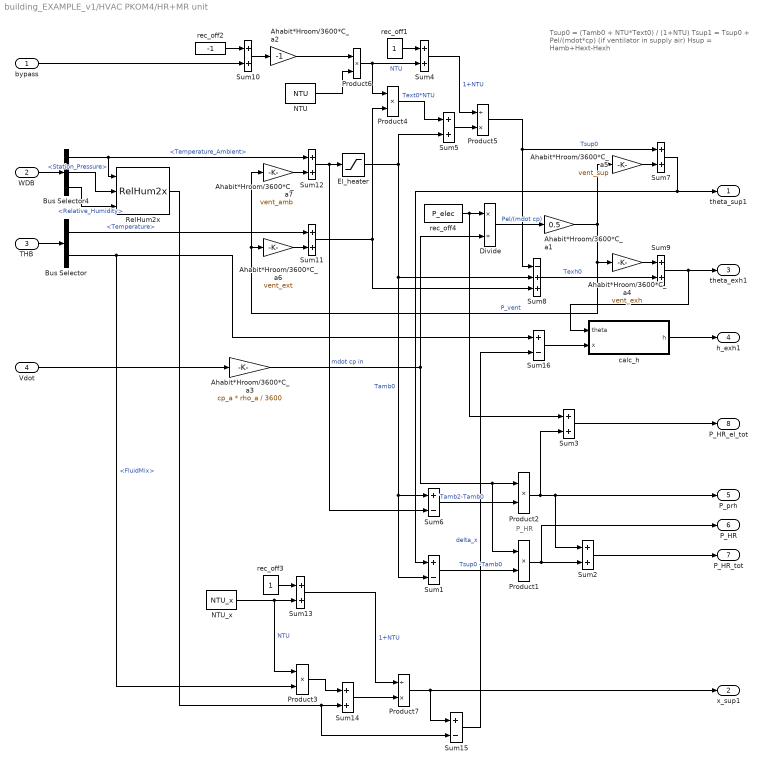
== system building_EXAMPLE_v1/HVAC PKOM4/HR+MR unit ==
  note: Tsup0 = (Tamb0 + NTU*Text0) / (1+NTU)
      | Tsup1 = Tsup0 + Pel/(mdot*cp)  (if ventilator in supply air)
      | Hsup = Hamb+Hext-Hexh
  note: P_HR
  bypass : Inport
  WDB : Inport  Port=2
  THB : Inport  Port=3
  Vdot : Inport  Port=4
  Ahabit*Hroom/3600*C_a1 : Gain  Gain=0.5  SaturateOnIntegerOverflow=on  OutDataTypeStr=Inherit: Same as input  ParamDataTypeStr=Inherit: Same as input
  Ahabit*Hroom/3600*C_a2 : Gain  Gain=-1  SaturateOnIntegerOverflow=on  OutDataTypeStr=Inherit: Same as input  ParamDataTypeStr=Inherit: Same as input
  Ahabit*Hroom/3600*C_a3 : Gain  Gain=cp_a * rho_a / 3600  SaturateOnIntegerOverflow=on  OutDataTypeStr=Inherit: Same as input  ParamDataTypeStr=Inherit: Same as input
  Ahabit*Hroom/3600*C_a4 : Gain  Gain=vent_exh  SaturateOnIntegerOverflow=on  OutDataTypeStr=Inherit: Same as input  ParamDataTypeStr=Inherit: Same as input
  Ahabit*Hroom/3600*C_a5 : Gain  Gain=vent_sup  SaturateOnIntegerOverflow=on  OutDataTypeStr=Inherit: Same as input  ParamDataTypeStr=Inherit: Same as input
  Ahabit*Hroom/3600*C_a6 : Gain  Gain=vent_ext  SaturateOnIntegerOverflow=on  OutDataTypeStr=Inherit: Same as input  ParamDataTypeStr=Inherit: Same as input
  Ahabit*Hroom/3600*C_a7 : Gain  Gain=vent_amb  SaturateOnIntegerOverflow=on  OutDataTypeStr=Inherit: Same as input  ParamDataTypeStr=Inherit: Same as input
  Bus Selector : BusSelector  OutputSignals=Temperature,FluidMix
  Bus Selector4 : BusSelector  OutputSignals=Temperature_Ambient,Station_Pressure,Relative_Humidity
  Divide : Product  Inputs=*/
  El_heater : Saturate  UpperLimit=inf  LowerLimit=low_lim
  NTU : Constant  Value=NTU
  NTU_x : Constant  Value=NTU_x
  Product{1..4,6} (5 alike) : Product  SaturateOnIntegerOverflow=on  InputSameDT=on  OutDataTypeStr=Inherit: Same as first input
  Product5 : Product  Inputs=/*  SaturateOnIntegerOverflow=on  InputSameDT=on  OutDataTypeStr=Inherit: Same as first input
  Product7 : Product  Inputs=/*  SaturateOnIntegerOverflow=on  InputSameDT=on  OutDataTypeStr=Inherit: Same as first input
  RelHum2x : carnot/Basic/Material_Properties/RelHum2x
  Sum{1,6,15..16} (4 alike) : Sum  Inputs=+-  SaturateOnIntegerOverflow=on  InputSameDT=on  OutDataTypeStr=Inherit: Same as first input
  Sum{4..5,7,9..14} (9 alike) : Sum  Inputs=2  SaturateOnIntegerOverflow=on  InputSameDT=on  OutDataTypeStr=Inherit: Same as first input
  Sum2 : Sum  SaturateOnIntegerOverflow=on  InputSameDT=on  OutDataTypeStr=Inherit: Same as first input
  Sum3 : Sum  SaturateOnIntegerOverflow=on  InputSameDT=on  OutDataTypeStr=Inherit: Same as first input
  Sum8 : Sum  Inputs=-++  SaturateOnIntegerOverflow=on  InputSameDT=on  OutDataTypeStr=Inherit: Same as first input
  calc_h : Subsystem
  rec_off1 : Constant
  rec_off2 : Constant  Value=-1
  rec_off3 : Constant
  rec_off4 : Constant  Value=P_elec
  theta_sup1 : Outport
  x_sup1 : Outport  Port=2
  theta_exh1 : Outport  Port=3
  h_exh1 : Outport  Port=4
  P_prh : Outport  Port=5
  P_HR : Outport  Port=6
  P_HR_tot : Outport  Port=7
  P_HR_el_tot : Outport  Port=8
  wires:
  Bus Selector4/1 -> RelHum2x/1, Sum12/1  "<Temperature_Ambient>"
  Ahabit*Hroom/3600*C_a7/1 -> Sum12/2
  Bus Selector/1 -> Sum11/1  "<Temperature>"
  Ahabit*Hroom/3600*C_a6/1 -> Sum11/2
  Bus Selector/2 -> Sum16/1, Product3/2  "<FluidMix>"
  calc_h/1(h) -> h_exh1/1
  Ahabit*Hroom/3600*C_a5/1 -> Sum7/2
  Ahabit*Hroom/3600*C_a4/1 -> Sum9/1
  THB/1 -> Bus Selector/1
  Sum12/1 -> Sum6/2, El_heater/1
  WDB/1 -> Bus Selector4/1
  Sum10/1 -> Ahabit*Hroom/3600*C_a2/1
  bypass/1 -> Sum10/2
  rec_off2/1 -> Sum10/1
  Ahabit*Hroom/3600*C_a2/1 -> Product6/1
  Ahabit*Hroom/3600*C_a3/1 -> Product1/1, Product2/1, Divide/2  "mdot cp in"
  Sum8/1 -> Sum9/2  "Texh0"
  Ahabit*Hroom/3600*C_a1/1 -> Ahabit*Hroom/3600*C_a4/1, Ahabit*Hroom/3600*C_a6/1, Ahabit*Hroom/3600*C_a7/1, Ahabit*Hroom/3600*C_a5/1  "P_vent"
  rec_off4/1 -> Divide/1, Sum3/1
  Divide/1 -> Ahabit*Hroom/3600*C_a1/1  "Pel/(mdot cp)"
  Product5/1 -> Sum8/1, Sum7/1  "Tsup0"
  Sum5/1 -> Product5/2
  rec_off1/1 -> Sum4/1
  Product4/1 -> Sum5/1  "Text0*NTU"
  Sum4/1 -> Product5/1  "1+NTU"
  NTU/1 -> Product6/2
  Product6/1 -> Sum4/2, Product4/1  "NTU"
  Sum3/1 -> P_HR_el_tot/1
  Sum2/1 -> P_HR_tot/1
  Product1/1 -> P_HR/1, Sum2/2
  Sum1/1 -> Product1/2  "Tsup0 -Tamb0"
  Product2/1 -> Sum3/2, Sum2/1, P_prh/1
  El_heater/1 -> Sum8/2, Sum1/2, Sum6/1, Sum5/2  "Tamb0"
  Sum7/1 -> Sum1/1, theta_sup1/1
  Vdot/1 -> Ahabit*Hroom/3600*C_a3/1
  Sum11/1 -> Product4/2, Sum8/3
  Sum9/1 -> theta_exh1/1, calc_h/1(theta)
  Sum6/1 -> Product2/2  "Tamb2-Tamb0"
  RelHum2x/1 -> Sum15/2, Sum14/2
  Bus Selector4/2 -> RelHum2x/2  "<Station_Pressure>"
  Bus Selector4/3 -> RelHum2x/3  "<Relative_Humidity>"
  rec_off3/1 -> Sum13/1
  Sum13/1 -> Product7/1  "1+NTU"
  NTU_x/1 -> Product3/1, Sum13/2  "NTU"
  Product3/1 -> Sum14/1
  Sum14/1 -> Product7/2
  Product7/1 -> x_sup1/1, Sum15/1
  Sum15/1 -> Sum16/2  "delta_x"
  Sum16/1 -> calc_h/2(x)

== system building_EXAMPLE_v1/HVAC PKOM4/Subsystem4 ==
  note: (kg/kg)
  note: (kg/s)
  note: (kg/s)
  note: (kg/s)
  mdot_air : Inport
  x_in : Inport  Port=2
  Demux3 : Demux  Outputs=2
  Fcn2 : Fcn  Expr=u / (1+u)
  Fcn3 : Fcn  Expr=u / (1+u)
  Product5 : Product  SaturateOnIntegerOverflow=on  InputSameDT=on  OutDataTypeStr=Inherit: Same as first input
  Product6 : Product  SaturateOnIntegerOverflow=on  InputSameDT=on  OutDataTypeStr=Inherit: Same as first input
  mdot_H2O : Outport  InitialOutput=0
  mdot_CO2 : Outport  Port=2  InitialOutput=0
  wires:
  Product5/1 -> mdot_H2O/1
  Product6/1 -> mdot_CO2/1
  mdot_air/1 -> Product5/1, Product6/1  "mdot_air >=0"
  Fcn3/1 -> Product6/2
  x_in/1 -> Demux3/1
  Demux3/1 -> Fcn2/1  "x_H2O_in"
  Demux3/2 -> Fcn3/1  "x_CO2_in"
  Fcn2/1 -> Product5/2

== system building_EXAMPLE_v1/HVAC PKOM4/controller summer bypass ==
  Troom : Inport
  WDB : Inport  Port=2
  Bus Selector4 : BusSelector  OutputSignals=Temperature_Ambient
  Data Type Conversion : DataTypeConversion  OutDataTypeStr=double
  Logical Operator : Logic  AllPortsSameDT=off  OutDataTypeStr=boolean
  Sum1 : Sum  Inputs=|++
  Tamb+deltatheta_amb < Troom : RelationalOperator  Operator=<  OutDataTypeStr=boolean  RndMeth=Simplest
  Troom > setpoint_bypass : RelationalOperator  OutDataTypeStr=boolean  RndMeth=Simplest
  deltatheta_amb : Constant  Value=hvac.controller.bypass.deltatheta_amb
  setpoint_bypass : Constant  Value=hvac.controller.setpoint_bypass
  temp sensor : simulink_extras/Additional Linear/Transfer Fcn (with initial outputs)  N=[1]  D=[hvac.controller.bypass.theta_amb_mean 1]  Y0=0  U0=0
  control bypass : Outport
  wires:
  Troom/1 -> Troom > setpoint_bypass/1, Tamb+deltatheta_amb < Troom/2
  Tamb+deltatheta_amb < Troom/1 -> Logical Operator/2
  Troom > setpoint_bypass/1 -> Logical Operator/1
  setpoint_bypass/1 -> Troom > setpoint_bypass/2
  Sum1/1 -> Tamb+deltatheta_amb < Troom/1
  deltatheta_amb/1 -> Sum1/2
  Bus Selector4/1 -> temp sensor/1  "<Temperature_Ambient>"
  WDB/1 -> Bus Selector4/1
  Logical Operator/1 -> Data Type Conversion/1
  temp sensor/1 -> Sum1/1
  Data Type Conversion/1 -> control bypass/1

== system building_EXAMPLE_v1/HVAC PKOM4/electrical heater 1 ==
  temperature room : Inport
  " " : Constant  Value=0
  "   " : Constant  Value=zeros(1,15)
  Bus Selector5 : BusSelector  OutputSignals=Ts
  Constant 3 : Constant  Value=theta_r_t  VectorParams1D=off
  Constant 9 : Constant  Value=theta_r_t_low  VectorParams1D=off
  Mux1 : Mux  Inputs=[1 1 15 1 1]
  PID_1 : simulink/Continuous/PID Controller  Controller=PI  TimeDomain=Continuous-time  SampleTime=-1  IntegratorMethod=Forward Euler  FilterMethod=Forward Euler  Form=Ideal  UseFilter=on  ControllerParametersSource=internal  P=Kp  I=(1/(Tn*60))  D=0  N=100  InitialConditionSource=internal  InitialConditionForIntegrator=0  InitialConditionForFilter=0  ExternalReset=none  LimitOutput=on  UpperSaturationLimit=1  LowerSaturationLimit=0  LinearizeAsGain=off  AntiWindupMode=clamping  Kb=1  TrackingMode=off  Kt=1  PParamMin=[]  PParamMax=[]  IParamMin=[]  IParamMax=[]  DParamMin=[]  DParamMax=[]  NParamMin=[]  NParamMax=[]  KbParamMin=[]  KbParamMax=[]  KtParamMin=[]  KtParamMax=[]  POutMin=[]  POutMax=[]  IOutMin=[]  IOutMax=[]  DOutMin=[]  DOutMax=[]  NOutMin=[]  NOutMax=[]  KbOutMin=[]  KbOutMax=[]  KtOutMin=[]  KtOutMax=[]  IntegratorOutMin=[]  IntegratorOutMax=[]  FilterOutMin=[]  FilterOutMax=[]  SumOutMin=[]  SumOutMax=[]  SumI1OutMin=[]  SumI1OutMax=[]  SumI2OutMin=[]  SumI2OutMax=[]  SumI3OutMin=[]  SumI3OutMax=[]  SumDOutMin=[]  SumDOutMax=[]  SaturationOutMin=[]  SaturationOutMax=[]  IntegratorContinuousStateAttributes=''  IntegratorStateMustResolveToSignalObject=off  IntegratorRTWStateStorageClass=Auto  FilterContinuousStateAttributes=''  FilterStateMustResolveToSignalObject=off  FilterRTWStateStorageClass=Auto  DifferentiatorICPrevScaledInput=0  DifferentiatorOutMin=[]  DifferentiatorOutMax=[]
  Sum13 : Sum  Inputs=|+-
  Switch : Switch  Criteria=u2 ~= 0
  Transfer Fcn (with initial states) : Subsystem  mask(Transfer Function with Initial States){N=[1], D=[timeconstant_heater  1], X0=0}
      mask prompts: N "Numerator:"; D "Denominator:"; X0 "Initial conditions:"
      mask help: Vector expressions for numerator, and denominator. Coefficients are in descending powers of s.
      mask init:
      | [A,B,C,Dd]=tf2ss(N,D);if (isempty(X0));[m,n]=size(A);X0=zeros(1,m); end;
      mask Help: Specify the initial states for the transfer function.  The state ordering is determined by the m-file tf2ss.  There is no unique mapping of the states in a transfer function to states in a state-space representation.  However, tf2ss will consistently use the same mapping for a given transfer function.
      mask Display: dpoly(N,D,'s')
  Transfer Fcn (with initial states)6 : Subsystem  mask(Transfer Function with Initial States){N=[1], D=[60  1], X0=0}
      mask prompts: N "Numerator:"; D "Denominator:"; X0 "Initial conditions:"
      mask help: Vector expressions for numerator, and denominator. Coefficients are in descending powers of s.
      mask init:
      | [A,B,C,Dd]=tf2ss(N,D);if (isempty(X0));[m,n]=size(A);X0=zeros(1,m); end;
      mask Help: Specify the initial states for the transfer function.  The state ordering is determined by the m-file tf2ss.  There is no unique mapping of the states in a transfer function to states in a state-space representation.  However, tf2ss will consistently use the same mapping for a given transfer function.
      mask Display: dpoly(N,D,'s')
  conv : Gain  Gain=1-part_rad  SaturateOnIntegerOverflow=on  OutDataTypeStr=Inherit: Same as input  ParamDataTypeStr=Inherit: Same as input
  heater : Product
  maximal power : Constant  Value=max_power
  rad : Gain  Gain=part_rad  SaturateOnIntegerOverflow=on  OutDataTypeStr=Inherit: Same as input  ParamDataTypeStr=Inherit: Same as input
  time profile : carnot/Load/General/Repeating_Profile  period=sum(control_time_duration)  rep_seq_t=control_time_values  rep_seq_d=control_time_duration  rep_seq_y=control_time_output
  "[S]" : Outport
  Pel : Outport  Port=2
  wires:
  time profile/1 -> Switch/2
  Switch/1 -> Sum13/1
  Constant 9/1 -> Switch/3
  Constant 3/1 -> Switch/1
  Transfer Fcn (with initial states)/1(Out1) -> Mux1/4, rad/1, conv/1
  Bus Selector5/1 -> Sum13/2  "<Ts>"
  Sum13/1 -> Transfer Fcn (with initial states)6/1(In1)
  heater/1 -> Transfer Fcn (with initial states)/1(In1), Pel/1
  "   "/1 -> Mux1/3
  rad/1 -> Mux1/2
  temperature room/1 -> Bus Selector5/1
  maximal power/1 -> heater/2
  conv/1 -> Mux1/1
  Mux1/1 -> "[S]"/1
  " "/1 -> Mux1/5
  PID_1/1 -> heater/1
  Transfer Fcn (with initial states)6/1(Out1) -> PID_1/1

== system building_EXAMPLE_v1/HVAC PKOM4/electrical heater 2 ==
  temperature room : Inport
  " " : Constant  Value=0
  "   " : Constant  Value=zeros(1,15)
  Bus Selector5 : BusSelector  OutputSignals=Ts
  Constant 3 : Constant  Value=theta_r_t  VectorParams1D=off
  Constant 9 : Constant  Value=theta_r_t_low  VectorParams1D=off
  Mux1 : Mux  Inputs=[1 1 15 1 1]
  PID_1 : simulink/Continuous/PID Controller  Controller=PI  TimeDomain=Continuous-time  SampleTime=-1  IntegratorMethod=Forward Euler  FilterMethod=Forward Euler  Form=Ideal  UseFilter=on  ControllerParametersSource=internal  P=Kp  I=(1/(Tn*60))  D=0  N=100  InitialConditionSource=internal  InitialConditionForIntegrator=0  InitialConditionForFilter=0  ExternalReset=none  LimitOutput=on  UpperSaturationLimit=1  LowerSaturationLimit=0  LinearizeAsGain=off  AntiWindupMode=clamping  Kb=1  TrackingMode=off  Kt=1  PParamMin=[]  PParamMax=[]  IParamMin=[]  IParamMax=[]  DParamMin=[]  DParamMax=[]  NParamMin=[]  NParamMax=[]  KbParamMin=[]  KbParamMax=[]  KtParamMin=[]  KtParamMax=[]  POutMin=[]  POutMax=[]  IOutMin=[]  IOutMax=[]  DOutMin=[]  DOutMax=[]  NOutMin=[]  NOutMax=[]  KbOutMin=[]  KbOutMax=[]  KtOutMin=[]  KtOutMax=[]  IntegratorOutMin=[]  IntegratorOutMax=[]  FilterOutMin=[]  FilterOutMax=[]  SumOutMin=[]  SumOutMax=[]  SumI1OutMin=[]  SumI1OutMax=[]  SumI2OutMin=[]  SumI2OutMax=[]  SumI3OutMin=[]  SumI3OutMax=[]  SumDOutMin=[]  SumDOutMax=[]  SaturationOutMin=[]  SaturationOutMax=[]  IntegratorContinuousStateAttributes=''  IntegratorStateMustResolveToSignalObject=off  IntegratorRTWStateStorageClass=Auto  FilterContinuousStateAttributes=''  FilterStateMustResolveToSignalObject=off  FilterRTWStateStorageClass=Auto  DifferentiatorICPrevScaledInput=0  DifferentiatorOutMin=[]  DifferentiatorOutMax=[]
  Sum13 : Sum  Inputs=|+-
  Switch : Switch  Criteria=u2 ~= 0
  Transfer Fcn (with initial states) : Subsystem  mask(Transfer Function with Initial States){N=[1], D=[timeconstant_heater  1], X0=0}
      mask prompts: N "Numerator:"; D "Denominator:"; X0 "Initial conditions:"
      mask help: Vector expressions for numerator, and denominator. Coefficients are in descending powers of s.
      mask init:
      | [A,B,C,Dd]=tf2ss(N,D);if (isempty(X0));[m,n]=size(A);X0=zeros(1,m); end;
      mask Help: Specify the initial states for the transfer function.  The state ordering is determined by the m-file tf2ss.  There is no unique mapping of the states in a transfer function to states in a state-space representation.  However, tf2ss will consistently use the same mapping for a given transfer function.
      mask Display: dpoly(N,D,'s')
  Transfer Fcn (with initial states)6 : Subsystem  mask(Transfer Function with Initial States){N=[1], D=[60  1], X0=0}
      mask prompts: N "Numerator:"; D "Denominator:"; X0 "Initial conditions:"
      mask help: Vector expressions for numerator, and denominator. Coefficients are in descending powers of s.
      mask init:
      | [A,B,C,Dd]=tf2ss(N,D);if (isempty(X0));[m,n]=size(A);X0=zeros(1,m); end;
      mask Help: Specify the initial states for the transfer function.  The state ordering is determined by the m-file tf2ss.  There is no unique mapping of the states in a transfer function to states in a state-space representation.  However, tf2ss will consistently use the same mapping for a given transfer function.
      mask Display: dpoly(N,D,'s')
  conv : Gain  Gain=1-part_rad  SaturateOnIntegerOverflow=on  OutDataTypeStr=Inherit: Same as input  ParamDataTypeStr=Inherit: Same as input
  heater : Product
  maximal power : Constant  Value=max_power
  rad : Gain  Gain=part_rad  SaturateOnIntegerOverflow=on  OutDataTypeStr=Inherit: Same as input  ParamDataTypeStr=Inherit: Same as input
  time profile : carnot/Load/General/Repeating_Profile  period=sum(control_time_duration)  rep_seq_t=control_time_values  rep_seq_d=control_time_duration  rep_seq_y=control_time_output
  "[S]" : Outport
  Pel : Outport  Port=2
  wires:
  Transfer Fcn (with initial states)6/1(Out1) -> PID_1/1
  PID_1/1 -> heater/1
  " "/1 -> Mux1/5
  Mux1/1 -> "[S]"/1
  conv/1 -> Mux1/1
  maximal power/1 -> heater/2
  temperature room/1 -> Bus Selector5/1
  rad/1 -> Mux1/2
  "   "/1 -> Mux1/3
  heater/1 -> Pel/1, Transfer Fcn (with initial states)/1(In1)
  Sum13/1 -> Transfer Fcn (with initial states)6/1(In1)
  Bus Selector5/1 -> Sum13/2  "<Ts>"
  Transfer Fcn (with initial states)/1(Out1) -> conv/1, rad/1, Mux1/4
  Constant 3/1 -> Switch/1
  Constant 9/1 -> Switch/3
  Switch/1 -> Sum13/1
  time profile/1 -> Switch/2
